simulink model "Tank2"  (R2016a)
settings: Solver=ode45  StartTime=0.0  StopTime=1000  RelTol=1e-3
undefined symbols (not defined in the file): b
libraries: TTLibrary x2
settings Model: Creator=blindner  LastModifiedBy=blindner
settings DataIOCC: LimitDataPoints=on  SaveFormat=Array  SaveOutput=off  SaveTime=off
settings DebuggingCC: SolverPrmCheckMsg=warning
settings HardwareCC: ProdBitPerPointer=32  ProdLargestAtomicFloat=None  ProdIntDivRoundTo=Undefined  ProdEndianess=Unspecified  ProdWordSize=32  ProdHWDeviceType=32-bit Generic
settings ModelReferenceCC: PropagateSignalLabelsOutOfModel=off
settings ConfigComp: CovModelRefEnable=Off  CovSFcnEnable=off

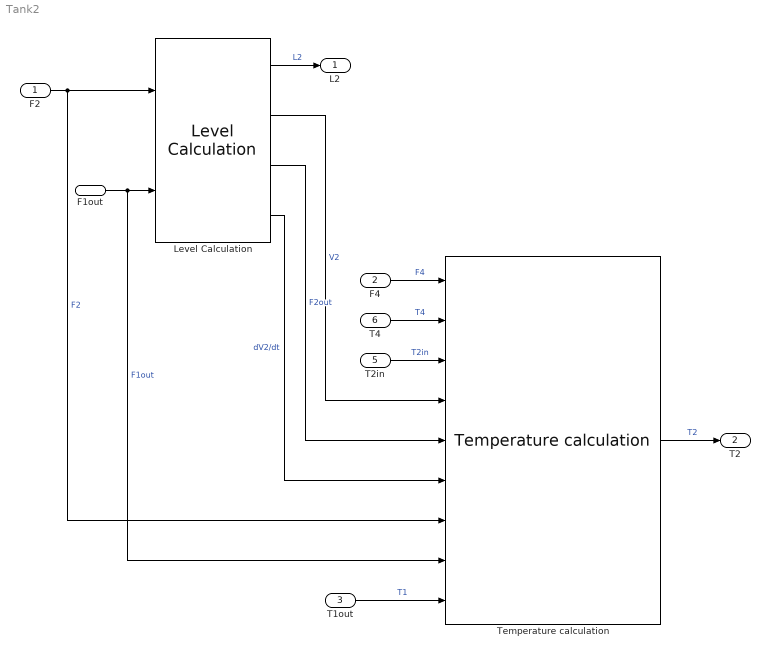
== system Tank2 ==
  F2 : Inport  OutDataTypeStr=double  PortDimensions=1  SampleTime=0
  F4 : Inport  Port=2  OutDataTypeStr=double  PortDimensions=1  SampleTime=0
  T1out : Inport  Port=3  OutDataTypeStr=double  PortDimensions=1  SampleTime=0
  F1out : Inport  Port=4  OutDataTypeStr=double  PortDimensions=1  SampleTime=0
  T2in : Inport  Port=5  OutDataTypeStr=double  PortDimensions=1  SampleTime=0
  T4 : Inport  Port=6  OutDataTypeStr=double  PortDimensions=1  SampleTime=0
  Level Calculation : TTLibrary/Level Calculation  kl=kl  Area=Area  Li=L2i  numIn=2
  Temperature calculation : TTLibrary/Temperature calculation  Ti=T2i  p=p  cp=cp  b=b  aHeat=aHeat  numIn=2
  L2 : Outport  OutDataTypeStr=double  PortDimensions=1  SampleTime=0
  "T2 " : Outport  Port=2  OutDataTypeStr=double  PortDimensions=1  SampleTime=0
  wires:
  F4/1 -> Temperature calculation/1  "F4"
  T1out/1 -> Temperature calculation/9  "T1"
  F1out/1 -> Level Calculation/2, Temperature calculation/8  "F1out"
  T2in/1 -> Temperature calculation/3  "T2in"
  T4/1 -> Temperature calculation/2  "T4"
  Level Calculation/1 -> L2/1  "L2"
  Level Calculation/3 -> Temperature calculation/5  "F2out"
  F2/1 -> Temperature calculation/7, Level Calculation/1  "F2"
  Temperature calculation/1 -> "T2 "/1  "T2"
  Level Calculation/4 -> Temperature calculation/6  "dV2/dt"
  Level Calculation/2 -> Temperature calculation/4  "V2"
